simulink library "INT_CoVMD_TrqDesCoord"  (R2016b)
settings: Solver=VariableStepAuto  StartTime=0.0  StopTime=10.0  RelTol=1e-3
settings Model: Creator=liutao  LastModifiedBy=liutao

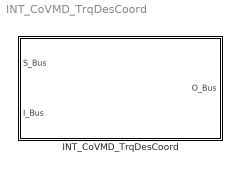
== system INT_CoVMD_TrqDesCoord ==
  INT_CoVMD_TrqDesCoord : Subsystem

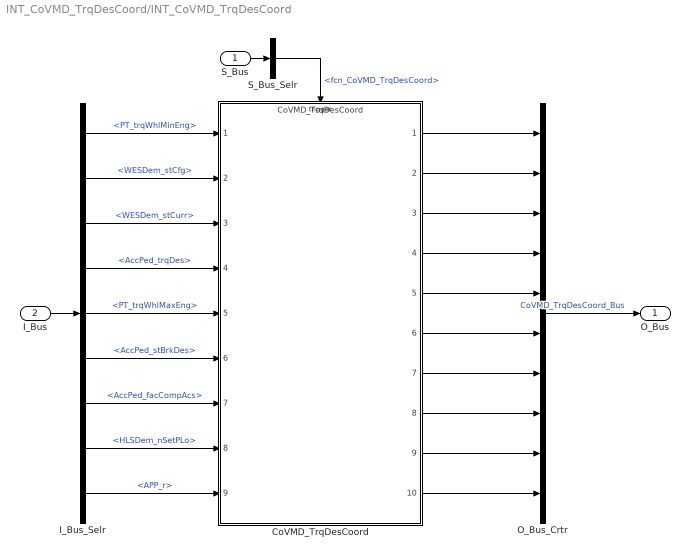
== system INT_CoVMD_TrqDesCoord/INT_CoVMD_TrqDesCoord ==
  S_Bus : Inport
  I_Bus : Inport  Port=2
  CoVMD_TrqDesCoord : ModelReference  ModelNameDialog=CoVMD_TrqDesCoord  SimulationMode=Normal  ModelReferenceVersion=1.37  TriggerPortName=function  TriggerPortTriggerType=function-call  TriggerPortStatesWhenEnabling=held
  I_Bus_Selr : BusSelector  OutputSignals=PT_trqWhlMinEng,WESDem_stCfg,WESDem_stCurr,AccPed_trqDes,PT_trqWhlMaxEng,AccPed_stBrkDes,AccPed_facCompAcs,HLSDem_nSetPLo,APP_r
  O_Bus_Crtr : BusCreator  Inputs=10
  S_Bus_Selr : BusSelector  OutputSignals=fcn_CoVMD_TrqDesCoord
  O_Bus : Outport
  wires:
  S_Bus_Selr/1 -> CoVMD_TrqDesCoord/Trigger  "<fcn_CoVMD_TrqDesCoord>"
  S_Bus/1 -> S_Bus_Selr/1
  I_Bus/1 -> I_Bus_Selr/1
  I_Bus_Selr/1 -> CoVMD_TrqDesCoord/1  "<PT_trqWhlMinEng>"
  I_Bus_Selr/2 -> CoVMD_TrqDesCoord/2  "<WESDem_stCfg>"
  I_Bus_Selr/3 -> CoVMD_TrqDesCoord/3  "<WESDem_stCurr>"
  I_Bus_Selr/4 -> CoVMD_TrqDesCoord/4  "<AccPed_trqDes>"
  I_Bus_Selr/5 -> CoVMD_TrqDesCoord/5  "<PT_trqWhlMaxEng>"
  I_Bus_Selr/6 -> CoVMD_TrqDesCoord/6  "<AccPed_stBrkDes>"
  I_Bus_Selr/7 -> CoVMD_TrqDesCoord/7  "<AccPed_facCompAcs>"
  I_Bus_Selr/8 -> CoVMD_TrqDesCoord/8  "<HLSDem_nSetPLo>"
  I_Bus_Selr/9 -> CoVMD_TrqDesCoord/9  "<APP_r>"
  O_Bus_Crtr/1 -> O_Bus/1  "CoVMD_TrqDesCoord_Bus"
  CoVMD_TrqDesCoord/1 -> O_Bus_Crtr/1
  CoVMD_TrqDesCoord/2 -> O_Bus_Crtr/2
  CoVMD_TrqDesCoord/3 -> O_Bus_Crtr/3
  CoVMD_TrqDesCoord/4 -> O_Bus_Crtr/4
  CoVMD_TrqDesCoord/5 -> O_Bus_Crtr/5
  CoVMD_TrqDesCoord/6 -> O_Bus_Crtr/6
  CoVMD_TrqDesCoord/7 -> O_Bus_Crtr/7
  CoVMD_TrqDesCoord/8 -> O_Bus_Crtr/8
  CoVMD_TrqDesCoord/9 -> O_Bus_Crtr/9
  CoVMD_TrqDesCoord/10 -> O_Bus_Crtr/10
